simulink model "SIMULACION_LTI_Aumentado"  (R2023b)
settings: Solver=VariableStepAuto  StartTime=0.0  StopTime=2  RelTol=1e-3
values from neighbouring files (symbols this model uses):
  Ld = 6.6e-3    (= 0.0066)    [C_Ids_comportamiento.m]
undefined symbols (not defined in the file or in its folder): b_eq, cts, J_eq, lambda_m, Lls, Lq, P_p, r, R_s, Rs_ref, Rts_amb, Tamb
settings Model: Creator=ignab  LastModifiedBy=ignab

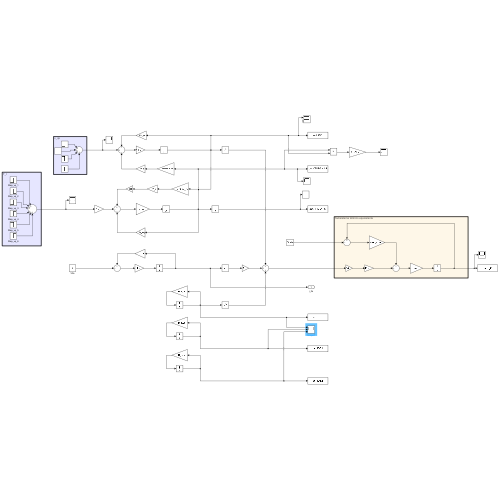
[thumbnail: Simulink's stored preview of the top-level diagram]
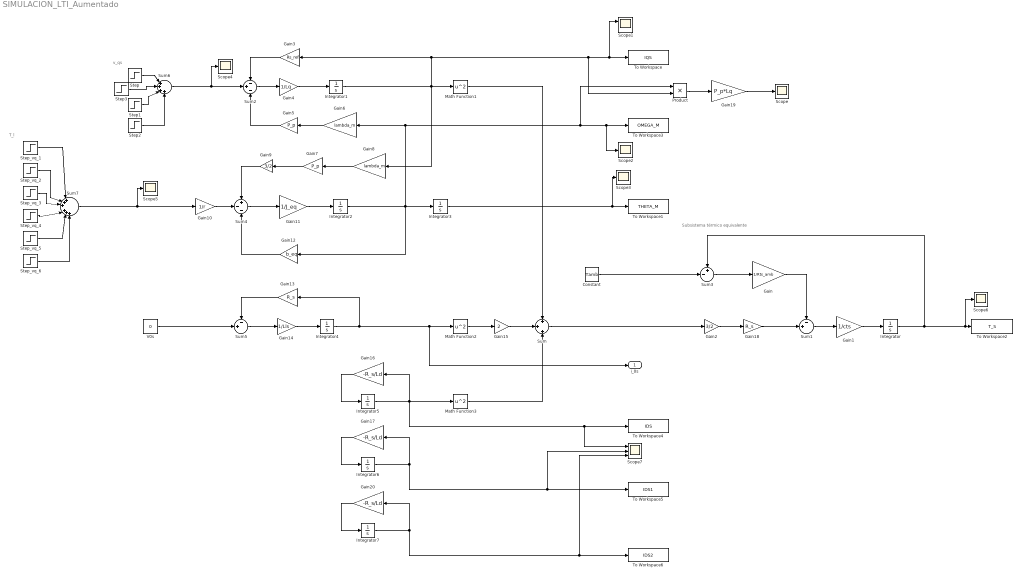
== system SIMULACION_LTI_Aumentado ==
  note: T_l
  note: v_qs
  note: Subsistema térmico equivalente
  Constant : Constant  Value=Tamb
  Gain : Gain  Gain=1/Rts_amb
  Gain1 : Gain  Gain=1/cts
  Gain10 : Gain  Gain=1/r
  Gain11 : Gain  Gain=1/J_eq
  Gain12 : Gain  Gain=b_eq
  Gain13 : Gain  Gain=R_s
  Gain14 : Gain  Gain=1/Lls
  Gain15 : Gain  Gain=2
  Gain16 : Gain  Gain=-R_s/Ld
  Gain17 : Gain  Gain=-R_s/Ld
  Gain18 : Gain  Gain=R_s
  Gain19 : Gain  Gain=P_p*Lq
  Gain2 : Gain  Gain=3/2
  Gain20 : Gain  Gain=-R_s/Ld
  Gain3 : Gain  Gain=Rs_ref
  Gain4 : Gain  Gain=1/Lq
  Gain5 : Gain  Gain=P_p
  Gain6 : Gain  Gain=lambda_m
  Gain7 : Gain  Gain=P_p
  Gain8 : Gain  Gain=lambda_m
  Gain9 : Gain  Gain=3/2
  Integrator{,1..5} (6 alike) : Integrator
  Integrator6 : Integrator  InitialCondition=0.5
  Integrator7 : Integrator  InitialCondition=-0.5
  Math Function1 : Math  Operator=square
  Math Function2 : Math  Operator=square
  Math Function3 : Math  Operator=square
  Product : Product
  Scope{,2..6} (6 alike) : Scope
  Scope1 : Scope  NumInputPorts=2
  Scope7 : Scope  NumInputPorts=3
  Step : Step  Time=0.1  After=19.596  SampleTime=0
  Step1 : Step  Time=1.1  After=-19.596  SampleTime=0
  Step2 : Step  Time=1.7  After=19.596  SampleTime=0
  Step3 : Step  Time=0.7  After=-19.596  SampleTime=0
  Step_vq_1 : Step  Time=0.3  After=6.28  SampleTime=0
  Step_vq_2 : Step  Time=0.5  After=-12.59  SampleTime=0
  Step_vq_3 : Step  Time=0.9  After=6.28  SampleTime=0
  Step_vq_4 : Step  Time=1.3  After=6.28  SampleTime=0
  Step_vq_5 : Step  Time=1.5  After=-12.59  SampleTime=0
  Step_vq_6 : Step  Time=1.9  After=6.28  SampleTime=0
  Sum : Sum  Inputs=+|+|+
  Sum1 : Sum  Inputs=-+|
  Sum2 : Sum  Inputs=-+-
  Sum3 : Sum  Inputs=+-|
  Sum4 : Sum  Inputs=+--
  Sum5 : Sum  Inputs=-+|
  Sum6 : Sum  Inputs=|++++
  Sum7 : Sum  Inputs=|+++|+++
  To Workspace : ToWorkspace  VariableName=IQS  SaveFormat=Timeseries  SampleTime=-1
      settings: Decimation=2
  To Workspace1 : ToWorkspace  VariableName=THETA_M  SaveFormat=Timeseries  SampleTime=-1
  To Workspace2 : ToWorkspace  VariableName=T_S  SaveFormat=Timeseries  SampleTime=-1
  To Workspace3 : ToWorkspace  VariableName=OMEGA_M  SaveFormat=Timeseries  SampleTime=-1
  To Workspace4 : ToWorkspace  VariableName=IDS  SaveFormat=Timeseries  SampleTime=-1
      settings: Decimation=2
  To Workspace5 : ToWorkspace  VariableName=IDS1  SaveFormat=Timeseries  SampleTime=-1
      settings: Decimation=2
  To Workspace6 : ToWorkspace  VariableName=IDS2  SaveFormat=Timeseries  SampleTime=-1
      settings: Decimation=2
  V0s : Constant  Value=0
  i_0s : Outport
  wires:
  Constant/1 -> Sum3/2
  Sum3/1 -> Gain/1
  Gain/1 -> Sum1/1
  Sum1/1 -> Gain1/1
  Gain1/1 -> Integrator/1
  Integrator/1 -> Scope6/1, To Workspace2/1, Sum3/1
  Sum6/1 -> Scope4/1, Sum2/2
  Gain5/1 -> Sum2/3
  Gain3/1 -> Sum2/1
  Sum2/1 -> Gain4/1
  Gain4/1 -> Integrator1/1
  Gain6/1 -> Gain5/1
  Integrator1/1 -> Product/2, Scope1/1, To Workspace/1, Gain3/1, Math Function1/1, Gain8/1
  Gain8/1 -> Gain7/1
  Gain7/1 -> Gain9/1
  Gain9/1 -> Sum4/1
  Gain12/1 -> Sum4/3
  Sum4/1 -> Gain11/1
  Gain11/1 -> Integrator2/1
  Integrator2/1 -> Integrator3/1, Gain12/1, Product/1, Scope2/1, To Workspace3/1, Gain6/1
  Gain10/1 -> Sum4/2
  Sum7/1 -> Scope5/1, Gain10/1
  Integrator4/1 -> i_0s/1, Math Function2/1, Gain13/1
  V0s/1 -> Sum5/2
  Sum5/1 -> Gain14/1
  Gain14/1 -> Integrator4/1
  Gain13/1 -> Sum5/1
  Integrator5/1 -> To Workspace4/1, Scope7/1, Gain16/1, Math Function3/1
  Math Function2/1 -> Gain15/1
  Math Function1/1 -> Sum/1
  Math Function3/1 -> Sum/3
  Sum/1 -> Gain2/1
  Gain2/1 -> Gain18/1
  Gain18/1 -> Sum1/2
  Integrator3/1 -> Scope3/1, To Workspace1/1
  Step2/1 -> Sum6/4
  Step/1 -> Sum6/1
  Step1/1 -> Sum6/3
  Step_vq_1/1 -> Sum7/1
  Step_vq_2/1 -> Sum7/2
  Step_vq_3/1 -> Sum7/3
  Step_vq_4/1 -> Sum7/4
  Step_vq_5/1 -> Sum7/5
  Step_vq_6/1 -> Sum7/6
  Product/1 -> Gain19/1
  Gain19/1 -> Scope/1
  Step3/1 -> Sum6/2
  Gain15/1 -> Sum/2
  Gain16/1 -> Integrator5/1
  Gain17/1 -> Integrator6/1
  Integrator6/1 -> To Workspace5/1, Scope7/2, Gain17/1
  Integrator7/1 -> To Workspace6/1, Scope7/3, Gain20/1
  Gain20/1 -> Integrator7/1
